simulink model "F16A_Physical"  (R2026a)
settings: Solver=VariableStepAuto
settings Model: DataDictionary=F16A_Physical.sldd  Creator=sdarshan  LastModifiedBy=sdarshan

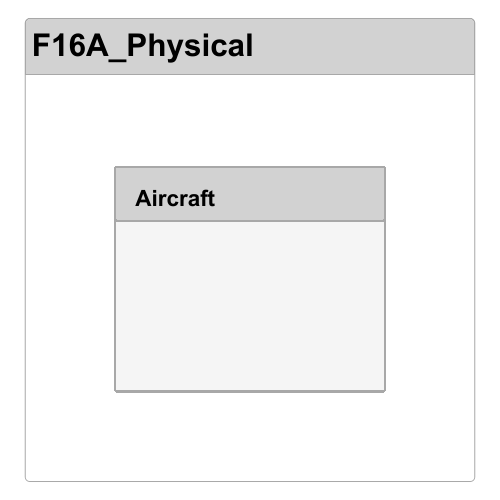
[thumbnail: Simulink's stored preview of the top-level diagram]
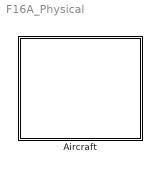
== system F16A_Physical ==
  Aircraft : Subsystem
      settings: PortSchema="{\"entries\":[{\"content\":{\"headerSize\":26,\"margin\":15,\"minimumSpacing\":25,\"sides\":[{\"content\":{},\"type\":\"ConnectorPlacement.EquallySpacedRectSide\",\"uuid\":\"d3b47e96-cd34-4867-b19b-ea6f12f6c501\"},{\"content\":{\"side\":\"RIGHT\"},\"type\":\"ConnectorPlacement.EquallySpacedRectSide\",\"uuid\":\"f31899f4-6bb1-4e7f-8ccb-f635929855f7\"},{\"content\":{\"side\":\"TOP\"},\"type\":\"ConnectorPlacement.EquallySpacedRectSide\",\"uuid\":\"ed462e8c-3ef6-416d-9984-fe5157ecba6e\"}]},\"type\":\"ConnectorPlacement.EquallySpacedConnector\",\"uuid\":\"a2af02c0-f4ca-4ebf-bacd-a22322d9a8f7\"}],\"packageUris\":[\"http://schema.mathworks.com/mf0/Connector/R2020b\"],\"version\":\"1.0\"}"

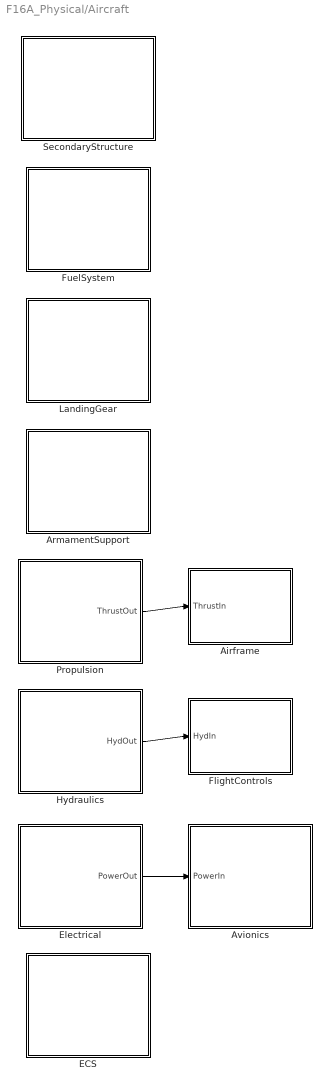
== system F16A_Physical/Aircraft ==
  Airframe : Subsystem  Variant=on  VariantControlMode=label  LabelModeActiveChoice=BlendedCrankedDelta
      settings: PortSchema="{\"entries\":[{\"content\":{\"headerSize\":38,\"margin\":15,\"minimumSpacing\":25,\"sides\":[{\"content\":{\"connectorIds\":[\"In1\"]},\"type\":\"ConnectorPlacement.EquallySpacedRectSide\",\"uuid\":\"40d085b4-dd18-4f67-ae88-aae7a5f696f7\"},{\"content\":{\"side\":\"RIGHT\"},\"type\":\"ConnectorPlacement.EquallySpacedRectSide\",\"uuid\":\"76a332b8-14bd-4810-ada5-8ab9c92fb4f5\"},{\"content\":{\"side\":\"TOP\"},\"type\":\"ConnectorPlacement.EquallySpacedRectSide\",\"uuid\":\"bda9a994-942d-4bdd-88a0-27c205fdec70\"}]},\"type\":\"ConnectorPlacement.EquallySpacedConnector\",\"uuid\":\"d2fd6e79-2d14-4962-a171-8f8cd008b298\"}],\"packageUris\":[\"http://schema.mathworks.com/mf0/Connector/R2020b\"],\"version\":\"1.0\"}"
  ArmamentSupport : Subsystem
      settings: PortSchema="{\"entries\":[{\"content\":{\"headerSize\":26,\"margin\":15,\"minimumSpacing\":25,\"sides\":[{\"content\":{},\"type\":\"ConnectorPlacement.EquallySpacedRectSide\",\"uuid\":\"d3b47e96-cd34-4867-b19b-ea6f12f6c501\"},{\"content\":{\"side\":\"RIGHT\"},\"type\":\"ConnectorPlacement.EquallySpacedRectSide\",\"uuid\":\"f31899f4-6bb1-4e7f-8ccb-f635929855f7\"},{\"content\":{\"side\":\"TOP\"},\"type\":\"ConnectorPlacement.EquallySpacedRectSide\",\"uuid\":\"ed462e8c-3ef6-416d-9984-fe5157ecba6e\"}]},\"type\":\"ConnectorPlacement.EquallySpacedConnector\",\"uuid\":\"a2af02c0-f4ca-4ebf-bacd-a22322d9a8f7\"}],\"packageUris\":[\"http://schema.mathworks.com/mf0/Connector/R2020b\"],\"version\":\"1.0\"}"
  Avionics : Subsystem
      settings: PortSchema="{\"entries\":[{\"content\":{\"headerSize\":26,\"margin\":15,\"minimumSpacing\":25,\"sides\":[{\"content\":{\"connectorIds\":[\"In1\"]},\"type\":\"ConnectorPlacement.EquallySpacedRectSide\",\"uuid\":\"d3b47e96-cd34-4867-b19b-ea6f12f6c501\"},{\"content\":{\"side\":\"RIGHT\"},\"type\":\"ConnectorPlacement.EquallySpacedRectSide\",\"uuid\":\"f31899f4-6bb1-4e7f-8ccb-f635929855f7\"},{\"content\":{\"side\":\"TOP\"},\"type\":\"ConnectorPlacement.EquallySpacedRectSide\",\"uuid\":\"ed462e8c-3ef6-416d-9984-fe5157ecba6e\"}]},\"type\":\"ConnectorPlacement.EquallySpacedConnector\",\"uuid\":\"a2af02c0-f4ca-4ebf-bacd-a22322d9a8f7\"}],\"packageUris\":[\"http://schema.mathworks.com/mf0/Connector/R2020b\"],\"version\":\"1.0\"}"
  ECS : Subsystem
      settings: PortSchema="{\"entries\":[{\"content\":{\"headerSize\":26,\"margin\":15,\"minimumSpacing\":25,\"sides\":[{\"content\":{},\"type\":\"ConnectorPlacement.EquallySpacedRectSide\",\"uuid\":\"d3b47e96-cd34-4867-b19b-ea6f12f6c501\"},{\"content\":{\"side\":\"RIGHT\"},\"type\":\"ConnectorPlacement.EquallySpacedRectSide\",\"uuid\":\"f31899f4-6bb1-4e7f-8ccb-f635929855f7\"},{\"content\":{\"side\":\"TOP\"},\"type\":\"ConnectorPlacement.EquallySpacedRectSide\",\"uuid\":\"ed462e8c-3ef6-416d-9984-fe5157ecba6e\"}]},\"type\":\"ConnectorPlacement.EquallySpacedConnector\",\"uuid\":\"a2af02c0-f4ca-4ebf-bacd-a22322d9a8f7\"}],\"packageUris\":[\"http://schema.mathworks.com/mf0/Connector/R2020b\"],\"version\":\"1.0\"}"
  Electrical : Subsystem
      settings: PortSchema="{\"entries\":[{\"content\":{\"headerSize\":26,\"margin\":15,\"minimumSpacing\":25,\"sides\":[{\"content\":{},\"type\":\"ConnectorPlacement.EquallySpacedRectSide\",\"uuid\":\"d3b47e96-cd34-4867-b19b-ea6f12f6c501\"},{\"content\":{\"connectorIds\":[\"Out1\"],\"side\":\"RIGHT\"},\"type\":\"ConnectorPlacement.EquallySpacedRectSide\",\"uuid\":\"f31899f4-6bb1-4e7f-8ccb-f635929855f7\"},{\"content\":{\"side\":\"TOP\"},\"type\":\"ConnectorPlacement.EquallySpacedRectSide\",\"uuid\":\"ed462e8c-3ef6-416d-9984-fe5157ecba6e\"}]},\"type\":\"ConnectorPlacement.EquallySpacedConnector\",\"uuid\":\"a2af02c0-f4ca-4ebf-bacd-a22322d9a8f7\"}],\"packageUris\":[\"http://schema.mathworks.com/mf0/Connector/R2020b\"],\"version\":\"1.0\"}"
  FlightControls : Subsystem  Variant=on  VariantControlMode=label  LabelModeActiveChoice=FlyByWire
      settings: PortSchema="{\"entries\":[{\"content\":{\"headerSize\":38,\"margin\":15,\"minimumSpacing\":25,\"sides\":[{\"content\":{\"connectorIds\":[\"In1\"]},\"type\":\"ConnectorPlacement.EquallySpacedRectSide\",\"uuid\":\"40d085b4-dd18-4f67-ae88-aae7a5f696f7\"},{\"content\":{\"side\":\"RIGHT\"},\"type\":\"ConnectorPlacement.EquallySpacedRectSide\",\"uuid\":\"76a332b8-14bd-4810-ada5-8ab9c92fb4f5\"},{\"content\":{\"side\":\"TOP\"},\"type\":\"ConnectorPlacement.EquallySpacedRectSide\",\"uuid\":\"bda9a994-942d-4bdd-88a0-27c205fdec70\"}]},\"type\":\"ConnectorPlacement.EquallySpacedConnector\",\"uuid\":\"d2fd6e79-2d14-4962-a171-8f8cd008b298\"}],\"packageUris\":[\"http://schema.mathworks.com/mf0/Connector/R2020b\"],\"version\":\"1.0\"}"
  FuelSystem : Subsystem
      settings: PortSchema="{\"entries\":[{\"content\":{\"headerSize\":26,\"margin\":15,\"minimumSpacing\":25,\"sides\":[{\"content\":{},\"type\":\"ConnectorPlacement.EquallySpacedRectSide\",\"uuid\":\"d3b47e96-cd34-4867-b19b-ea6f12f6c501\"},{\"content\":{\"side\":\"RIGHT\"},\"type\":\"ConnectorPlacement.EquallySpacedRectSide\",\"uuid\":\"f31899f4-6bb1-4e7f-8ccb-f635929855f7\"},{\"content\":{\"side\":\"TOP\"},\"type\":\"ConnectorPlacement.EquallySpacedRectSide\",\"uuid\":\"ed462e8c-3ef6-416d-9984-fe5157ecba6e\"}]},\"type\":\"ConnectorPlacement.EquallySpacedConnector\",\"uuid\":\"a2af02c0-f4ca-4ebf-bacd-a22322d9a8f7\"}],\"packageUris\":[\"http://schema.mathworks.com/mf0/Connector/R2020b\"],\"version\":\"1.0\"}"
  Hydraulics : Subsystem
      settings: PortSchema="{\"entries\":[{\"content\":{\"headerSize\":26,\"margin\":15,\"minimumSpacing\":25,\"sides\":[{\"content\":{},\"type\":\"ConnectorPlacement.EquallySpacedRectSide\",\"uuid\":\"d3b47e96-cd34-4867-b19b-ea6f12f6c501\"},{\"content\":{\"connectorIds\":[\"Out1\"],\"side\":\"RIGHT\"},\"type\":\"ConnectorPlacement.EquallySpacedRectSide\",\"uuid\":\"f31899f4-6bb1-4e7f-8ccb-f635929855f7\"},{\"content\":{\"side\":\"TOP\"},\"type\":\"ConnectorPlacement.EquallySpacedRectSide\",\"uuid\":\"ed462e8c-3ef6-416d-9984-fe5157ecba6e\"}]},\"type\":\"ConnectorPlacement.EquallySpacedConnector\",\"uuid\":\"a2af02c0-f4ca-4ebf-bacd-a22322d9a8f7\"}],\"packageUris\":[\"http://schema.mathworks.com/mf0/Connector/R2020b\"],\"version\":\"1.0\"}"
  LandingGear : Subsystem
      settings: PortSchema="{\"entries\":[{\"content\":{\"headerSize\":26,\"margin\":15,\"minimumSpacing\":25,\"sides\":[{\"content\":{},\"type\":\"ConnectorPlacement.EquallySpacedRectSide\",\"uuid\":\"d3b47e96-cd34-4867-b19b-ea6f12f6c501\"},{\"content\":{\"side\":\"RIGHT\"},\"type\":\"ConnectorPlacement.EquallySpacedRectSide\",\"uuid\":\"f31899f4-6bb1-4e7f-8ccb-f635929855f7\"},{\"content\":{\"side\":\"TOP\"},\"type\":\"ConnectorPlacement.EquallySpacedRectSide\",\"uuid\":\"ed462e8c-3ef6-416d-9984-fe5157ecba6e\"}]},\"type\":\"ConnectorPlacement.EquallySpacedConnector\",\"uuid\":\"a2af02c0-f4ca-4ebf-bacd-a22322d9a8f7\"}],\"packageUris\":[\"http://schema.mathworks.com/mf0/Connector/R2020b\"],\"version\":\"1.0\"}"
  Propulsion : Subsystem
      settings: PortSchema="{\"entries\":[{\"content\":{\"headerSize\":26,\"margin\":15,\"minimumSpacing\":25,\"sides\":[{\"content\":{},\"type\":\"ConnectorPlacement.EquallySpacedRectSide\",\"uuid\":\"d3b47e96-cd34-4867-b19b-ea6f12f6c501\"},{\"content\":{\"connectorIds\":[\"Out1\"],\"side\":\"RIGHT\"},\"type\":\"ConnectorPlacement.EquallySpacedRectSide\",\"uuid\":\"f31899f4-6bb1-4e7f-8ccb-f635929855f7\"},{\"content\":{\"side\":\"TOP\"},\"type\":\"ConnectorPlacement.EquallySpacedRectSide\",\"uuid\":\"ed462e8c-3ef6-416d-9984-fe5157ecba6e\"}]},\"type\":\"ConnectorPlacement.EquallySpacedConnector\",\"uuid\":\"a2af02c0-f4ca-4ebf-bacd-a22322d9a8f7\"}],\"packageUris\":[\"http://schema.mathworks.com/mf0/Connector/R2020b\"],\"version\":\"1.0\"}"
  SecondaryStructure : Subsystem
      settings: PortSchema="{\"entries\":[{\"content\":{\"headerSize\":26,\"margin\":15,\"minimumSpacing\":25,\"sides\":[{\"content\":{},\"type\":\"ConnectorPlacement.EquallySpacedRectSide\",\"uuid\":\"d3b47e96-cd34-4867-b19b-ea6f12f6c501\"},{\"content\":{\"side\":\"RIGHT\"},\"type\":\"ConnectorPlacement.EquallySpacedRectSide\",\"uuid\":\"f31899f4-6bb1-4e7f-8ccb-f635929855f7\"},{\"content\":{\"side\":\"TOP\"},\"type\":\"ConnectorPlacement.EquallySpacedRectSide\",\"uuid\":\"ed462e8c-3ef6-416d-9984-fe5157ecba6e\"}]},\"type\":\"ConnectorPlacement.EquallySpacedConnector\",\"uuid\":\"a2af02c0-f4ca-4ebf-bacd-a22322d9a8f7\"}],\"packageUris\":[\"http://schema.mathworks.com/mf0/Connector/R2020b\"],\"version\":\"1.0\"}"
  wires:
  Electrical/1(PowerOut) -> Avionics/1(PowerIn)
  Hydraulics/1(HydOut) -> FlightControls/1(HydIn)
  Propulsion/1(ThrustOut) -> Airframe/1(ThrustIn)

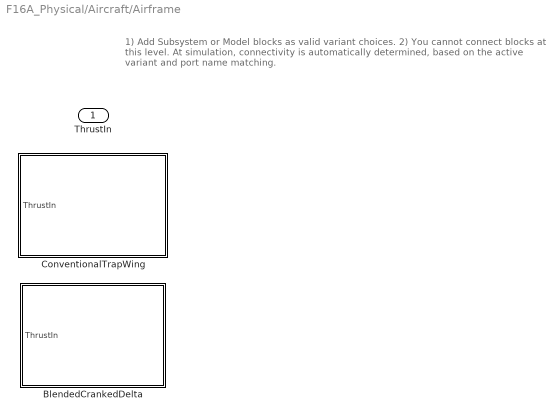
== system F16A_Physical/Aircraft/Airframe ==
  note: 1) Add Subsystem or Model blocks as valid variant choices.
      | 2) You cannot connect blocks at this level. At simulation, connectivity is automatically
      | determined, based on the active variant and port name matching.
  ThrustIn : Inport
  BlendedCrankedDelta : Subsystem  VariantControl=BlendedCrankedDelta
      settings: PortSchema="{\"entries\":[{\"content\":{\"headerSize\":26,\"margin\":15,\"minimumSpacing\":25,\"sides\":[{\"content\":{\"connectorIds\":[\"In1\"]},\"type\":\"ConnectorPlacement.EquallySpacedRectSide\",\"uuid\":\"d3b47e96-cd34-4867-b19b-ea6f12f6c501\"},{\"content\":{\"side\":\"RIGHT\"},\"type\":\"ConnectorPlacement.EquallySpacedRectSide\",\"uuid\":\"f31899f4-6bb1-4e7f-8ccb-f635929855f7\"},{\"content\":{\"side\":\"TOP\"},\"type\":\"ConnectorPlacement.EquallySpacedRectSide\",\"uuid\":\"ed462e8c-3ef6-416d-9984-fe5157ecba6e\"}]},\"type\":\"ConnectorPlacement.EquallySpacedConnector\",\"uuid\":\"a2af02c0-f4ca-4ebf-bacd-a22322d9a8f7\"}],\"packageUris\":[\"http://schema.mathworks.com/mf0/Connector/R2020b\"],\"version\":\"1.0\"}"
  ConventionalTrapWing : Subsystem  VariantControl=ConventionalTrapWing
      settings: PortSchema="{\"entries\":[{\"content\":{\"headerSize\":26,\"margin\":15,\"minimumSpacing\":25,\"sides\":[{\"content\":{\"connectorIds\":[\"In1\"]},\"type\":\"ConnectorPlacement.EquallySpacedRectSide\",\"uuid\":\"d3b47e96-cd34-4867-b19b-ea6f12f6c501\"},{\"content\":{\"side\":\"RIGHT\"},\"type\":\"ConnectorPlacement.EquallySpacedRectSide\",\"uuid\":\"f31899f4-6bb1-4e7f-8ccb-f635929855f7\"},{\"content\":{\"side\":\"TOP\"},\"type\":\"ConnectorPlacement.EquallySpacedRectSide\",\"uuid\":\"ed462e8c-3ef6-416d-9984-fe5157ecba6e\"}]},\"type\":\"ConnectorPlacement.EquallySpacedConnector\",\"uuid\":\"a2af02c0-f4ca-4ebf-bacd-a22322d9a8f7\"}],\"packageUris\":[\"http://schema.mathworks.com/mf0/Connector/R2020b\"],\"version\":\"1.0\"}"

== system F16A_Physical/Aircraft/ArmamentSupport ==

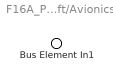
== system F16A_Physical/Aircraft/Avionics ==
  Bus Element In1 : Inport  PortName=PowerIn

== system F16A_Physical/Aircraft/ECS ==

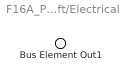
== system F16A_Physical/Aircraft/Electrical ==
  Bus Element Out1 : Outport  PortName=PowerOut

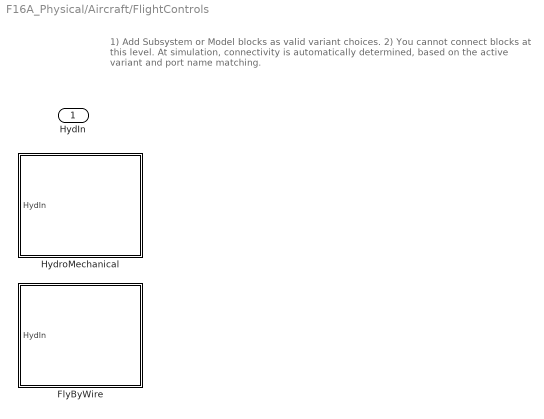
== system F16A_Physical/Aircraft/FlightControls ==
  note: 1) Add Subsystem or Model blocks as valid variant choices.
      | 2) You cannot connect blocks at this level. At simulation, connectivity is automatically
      | determined, based on the active variant and port name matching.
  HydIn : Inport
  FlyByWire : Subsystem  VariantControl=FlyByWire
      settings: PortSchema="{\"entries\":[{\"content\":{\"headerSize\":26,\"margin\":15,\"minimumSpacing\":25,\"sides\":[{\"content\":{\"connectorIds\":[\"In1\"]},\"type\":\"ConnectorPlacement.EquallySpacedRectSide\",\"uuid\":\"d3b47e96-cd34-4867-b19b-ea6f12f6c501\"},{\"content\":{\"side\":\"RIGHT\"},\"type\":\"ConnectorPlacement.EquallySpacedRectSide\",\"uuid\":\"f31899f4-6bb1-4e7f-8ccb-f635929855f7\"},{\"content\":{\"side\":\"TOP\"},\"type\":\"ConnectorPlacement.EquallySpacedRectSide\",\"uuid\":\"ed462e8c-3ef6-416d-9984-fe5157ecba6e\"}]},\"type\":\"ConnectorPlacement.EquallySpacedConnector\",\"uuid\":\"a2af02c0-f4ca-4ebf-bacd-a22322d9a8f7\"}],\"packageUris\":[\"http://schema.mathworks.com/mf0/Connector/R2020b\"],\"version\":\"1.0\"}"
  HydroMechanical : Subsystem  VariantControl=HydroMechanical
      settings: PortSchema="{\"entries\":[{\"content\":{\"headerSize\":26,\"margin\":15,\"minimumSpacing\":25,\"sides\":[{\"content\":{\"connectorIds\":[\"In1\"]},\"type\":\"ConnectorPlacement.EquallySpacedRectSide\",\"uuid\":\"d3b47e96-cd34-4867-b19b-ea6f12f6c501\"},{\"content\":{\"side\":\"RIGHT\"},\"type\":\"ConnectorPlacement.EquallySpacedRectSide\",\"uuid\":\"f31899f4-6bb1-4e7f-8ccb-f635929855f7\"},{\"content\":{\"side\":\"TOP\"},\"type\":\"ConnectorPlacement.EquallySpacedRectSide\",\"uuid\":\"ed462e8c-3ef6-416d-9984-fe5157ecba6e\"}]},\"type\":\"ConnectorPlacement.EquallySpacedConnector\",\"uuid\":\"a2af02c0-f4ca-4ebf-bacd-a22322d9a8f7\"}],\"packageUris\":[\"http://schema.mathworks.com/mf0/Connector/R2020b\"],\"version\":\"1.0\"}"

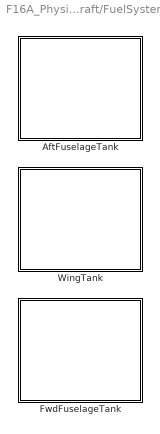
== system F16A_Physical/Aircraft/FuelSystem ==
  AftFuselageTank : Subsystem
      settings: PortSchema="{\"entries\":[{\"content\":{\"headerSize\":26,\"margin\":15,\"minimumSpacing\":25,\"sides\":[{\"content\":{},\"type\":\"ConnectorPlacement.EquallySpacedRectSide\",\"uuid\":\"d3b47e96-cd34-4867-b19b-ea6f12f6c501\"},{\"content\":{\"side\":\"RIGHT\"},\"type\":\"ConnectorPlacement.EquallySpacedRectSide\",\"uuid\":\"f31899f4-6bb1-4e7f-8ccb-f635929855f7\"},{\"content\":{\"side\":\"TOP\"},\"type\":\"ConnectorPlacement.EquallySpacedRectSide\",\"uuid\":\"ed462e8c-3ef6-416d-9984-fe5157ecba6e\"}]},\"type\":\"ConnectorPlacement.EquallySpacedConnector\",\"uuid\":\"a2af02c0-f4ca-4ebf-bacd-a22322d9a8f7\"}],\"packageUris\":[\"http://schema.mathworks.com/mf0/Connector/R2020b\"],\"version\":\"1.0\"}"
  FwdFuselageTank : Subsystem
      settings: PortSchema="{\"entries\":[{\"content\":{\"headerSize\":26,\"margin\":15,\"minimumSpacing\":25,\"sides\":[{\"content\":{},\"type\":\"ConnectorPlacement.EquallySpacedRectSide\",\"uuid\":\"d3b47e96-cd34-4867-b19b-ea6f12f6c501\"},{\"content\":{\"side\":\"RIGHT\"},\"type\":\"ConnectorPlacement.EquallySpacedRectSide\",\"uuid\":\"f31899f4-6bb1-4e7f-8ccb-f635929855f7\"},{\"content\":{\"side\":\"TOP\"},\"type\":\"ConnectorPlacement.EquallySpacedRectSide\",\"uuid\":\"ed462e8c-3ef6-416d-9984-fe5157ecba6e\"}]},\"type\":\"ConnectorPlacement.EquallySpacedConnector\",\"uuid\":\"a2af02c0-f4ca-4ebf-bacd-a22322d9a8f7\"}],\"packageUris\":[\"http://schema.mathworks.com/mf0/Connector/R2020b\"],\"version\":\"1.0\"}"
  WingTank : Subsystem
      settings: PortSchema="{\"entries\":[{\"content\":{\"headerSize\":26,\"margin\":15,\"minimumSpacing\":25,\"sides\":[{\"content\":{},\"type\":\"ConnectorPlacement.EquallySpacedRectSide\",\"uuid\":\"d3b47e96-cd34-4867-b19b-ea6f12f6c501\"},{\"content\":{\"side\":\"RIGHT\"},\"type\":\"ConnectorPlacement.EquallySpacedRectSide\",\"uuid\":\"f31899f4-6bb1-4e7f-8ccb-f635929855f7\"},{\"content\":{\"side\":\"TOP\"},\"type\":\"ConnectorPlacement.EquallySpacedRectSide\",\"uuid\":\"ed462e8c-3ef6-416d-9984-fe5157ecba6e\"}]},\"type\":\"ConnectorPlacement.EquallySpacedConnector\",\"uuid\":\"a2af02c0-f4ca-4ebf-bacd-a22322d9a8f7\"}],\"packageUris\":[\"http://schema.mathworks.com/mf0/Connector/R2020b\"],\"version\":\"1.0\"}"

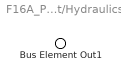
== system F16A_Physical/Aircraft/Hydraulics ==
  Bus Element Out1 : Outport  PortName=HydOut

== system F16A_Physical/Aircraft/LandingGear ==

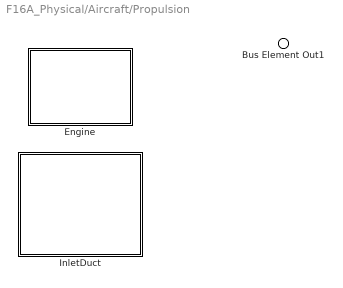
== system F16A_Physical/Aircraft/Propulsion ==
  Engine : Subsystem  Variant=on  VariantControlMode=label  LabelModeActiveChoice=F100_PW_200
      settings: PortSchema="{\"entries\":[{\"content\":{\"headerSize\":38,\"margin\":15,\"minimumSpacing\":25,\"sides\":[{\"content\":{},\"type\":\"ConnectorPlacement.EquallySpacedRectSide\",\"uuid\":\"40d085b4-dd18-4f67-ae88-aae7a5f696f7\"},{\"content\":{\"side\":\"RIGHT\"},\"type\":\"ConnectorPlacement.EquallySpacedRectSide\",\"uuid\":\"76a332b8-14bd-4810-ada5-8ab9c92fb4f5\"},{\"content\":{\"side\":\"TOP\"},\"type\":\"ConnectorPlacement.EquallySpacedRectSide\",\"uuid\":\"bda9a994-942d-4bdd-88a0-27c205fdec70\"}]},\"type\":\"ConnectorPlacement.EquallySpacedConnector\",\"uuid\":\"d2fd6e79-2d14-4962-a171-8f8cd008b298\"}],\"packageUris\":[\"http://schema.mathworks.com/mf0/Connector/R2020b\"],\"version\":\"1.0\"}"
  InletDuct : Subsystem
      settings: PortSchema="{\"entries\":[{\"content\":{\"headerSize\":26,\"margin\":15,\"minimumSpacing\":25,\"sides\":[{\"content\":{},\"type\":\"ConnectorPlacement.EquallySpacedRectSide\",\"uuid\":\"d3b47e96-cd34-4867-b19b-ea6f12f6c501\"},{\"content\":{\"side\":\"RIGHT\"},\"type\":\"ConnectorPlacement.EquallySpacedRectSide\",\"uuid\":\"f31899f4-6bb1-4e7f-8ccb-f635929855f7\"},{\"content\":{\"side\":\"TOP\"},\"type\":\"ConnectorPlacement.EquallySpacedRectSide\",\"uuid\":\"ed462e8c-3ef6-416d-9984-fe5157ecba6e\"}]},\"type\":\"ConnectorPlacement.EquallySpacedConnector\",\"uuid\":\"a2af02c0-f4ca-4ebf-bacd-a22322d9a8f7\"}],\"packageUris\":[\"http://schema.mathworks.com/mf0/Connector/R2020b\"],\"version\":\"1.0\"}"
  Bus Element Out1 : Outport  PortName=ThrustOut

== system F16A_Physical/Aircraft/SecondaryStructure ==

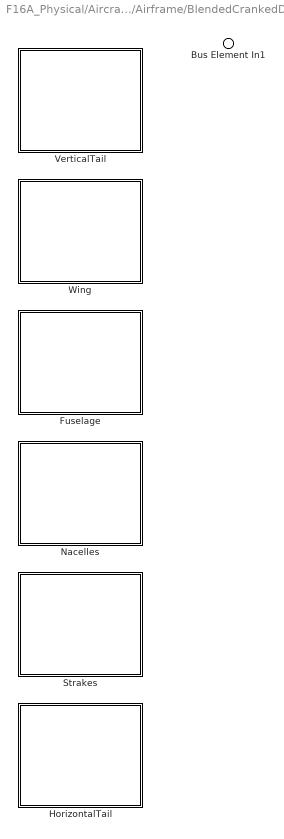
== system F16A_Physical/Aircraft/Airframe/BlendedCrankedDelta ==
  Bus Element In1 : Inport  PortName=ThrustIn
  Fuselage : Subsystem
      settings: PortSchema="{\"entries\":[{\"content\":{\"headerSize\":26,\"margin\":15,\"minimumSpacing\":25,\"sides\":[{\"content\":{},\"type\":\"ConnectorPlacement.EquallySpacedRectSide\",\"uuid\":\"d3b47e96-cd34-4867-b19b-ea6f12f6c501\"},{\"content\":{\"side\":\"RIGHT\"},\"type\":\"ConnectorPlacement.EquallySpacedRectSide\",\"uuid\":\"f31899f4-6bb1-4e7f-8ccb-f635929855f7\"},{\"content\":{\"side\":\"TOP\"},\"type\":\"ConnectorPlacement.EquallySpacedRectSide\",\"uuid\":\"ed462e8c-3ef6-416d-9984-fe5157ecba6e\"}]},\"type\":\"ConnectorPlacement.EquallySpacedConnector\",\"uuid\":\"a2af02c0-f4ca-4ebf-bacd-a22322d9a8f7\"}],\"packageUris\":[\"http://schema.mathworks.com/mf0/Connector/R2020b\"],\"version\":\"1.0\"}"
  HorizontalTail : Subsystem
      settings: PortSchema="{\"entries\":[{\"content\":{\"headerSize\":26,\"margin\":15,\"minimumSpacing\":25,\"sides\":[{\"content\":{},\"type\":\"ConnectorPlacement.EquallySpacedRectSide\",\"uuid\":\"d3b47e96-cd34-4867-b19b-ea6f12f6c501\"},{\"content\":{\"side\":\"RIGHT\"},\"type\":\"ConnectorPlacement.EquallySpacedRectSide\",\"uuid\":\"f31899f4-6bb1-4e7f-8ccb-f635929855f7\"},{\"content\":{\"side\":\"TOP\"},\"type\":\"ConnectorPlacement.EquallySpacedRectSide\",\"uuid\":\"ed462e8c-3ef6-416d-9984-fe5157ecba6e\"}]},\"type\":\"ConnectorPlacement.EquallySpacedConnector\",\"uuid\":\"a2af02c0-f4ca-4ebf-bacd-a22322d9a8f7\"}],\"packageUris\":[\"http://schema.mathworks.com/mf0/Connector/R2020b\"],\"version\":\"1.0\"}"
  Nacelles : Subsystem
      settings: PortSchema="{\"entries\":[{\"content\":{\"headerSize\":26,\"margin\":15,\"minimumSpacing\":25,\"sides\":[{\"content\":{},\"type\":\"ConnectorPlacement.EquallySpacedRectSide\",\"uuid\":\"d3b47e96-cd34-4867-b19b-ea6f12f6c501\"},{\"content\":{\"side\":\"RIGHT\"},\"type\":\"ConnectorPlacement.EquallySpacedRectSide\",\"uuid\":\"f31899f4-6bb1-4e7f-8ccb-f635929855f7\"},{\"content\":{\"side\":\"TOP\"},\"type\":\"ConnectorPlacement.EquallySpacedRectSide\",\"uuid\":\"ed462e8c-3ef6-416d-9984-fe5157ecba6e\"}]},\"type\":\"ConnectorPlacement.EquallySpacedConnector\",\"uuid\":\"a2af02c0-f4ca-4ebf-bacd-a22322d9a8f7\"}],\"packageUris\":[\"http://schema.mathworks.com/mf0/Connector/R2020b\"],\"version\":\"1.0\"}"
  Strakes : Subsystem
      settings: PortSchema="{\"entries\":[{\"content\":{\"headerSize\":26,\"margin\":15,\"minimumSpacing\":25,\"sides\":[{\"content\":{},\"type\":\"ConnectorPlacement.EquallySpacedRectSide\",\"uuid\":\"d3b47e96-cd34-4867-b19b-ea6f12f6c501\"},{\"content\":{\"side\":\"RIGHT\"},\"type\":\"ConnectorPlacement.EquallySpacedRectSide\",\"uuid\":\"f31899f4-6bb1-4e7f-8ccb-f635929855f7\"},{\"content\":{\"side\":\"TOP\"},\"type\":\"ConnectorPlacement.EquallySpacedRectSide\",\"uuid\":\"ed462e8c-3ef6-416d-9984-fe5157ecba6e\"}]},\"type\":\"ConnectorPlacement.EquallySpacedConnector\",\"uuid\":\"a2af02c0-f4ca-4ebf-bacd-a22322d9a8f7\"}],\"packageUris\":[\"http://schema.mathworks.com/mf0/Connector/R2020b\"],\"version\":\"1.0\"}"
  VerticalTail : Subsystem
      settings: PortSchema="{\"entries\":[{\"content\":{\"headerSize\":26,\"margin\":15,\"minimumSpacing\":25,\"sides\":[{\"content\":{},\"type\":\"ConnectorPlacement.EquallySpacedRectSide\",\"uuid\":\"d3b47e96-cd34-4867-b19b-ea6f12f6c501\"},{\"content\":{\"side\":\"RIGHT\"},\"type\":\"ConnectorPlacement.EquallySpacedRectSide\",\"uuid\":\"f31899f4-6bb1-4e7f-8ccb-f635929855f7\"},{\"content\":{\"side\":\"TOP\"},\"type\":\"ConnectorPlacement.EquallySpacedRectSide\",\"uuid\":\"ed462e8c-3ef6-416d-9984-fe5157ecba6e\"}]},\"type\":\"ConnectorPlacement.EquallySpacedConnector\",\"uuid\":\"a2af02c0-f4ca-4ebf-bacd-a22322d9a8f7\"}],\"packageUris\":[\"http://schema.mathworks.com/mf0/Connector/R2020b\"],\"version\":\"1.0\"}"
  Wing : Subsystem
      settings: PortSchema="{\"entries\":[{\"content\":{\"headerSize\":26,\"margin\":15,\"minimumSpacing\":25,\"sides\":[{\"content\":{},\"type\":\"ConnectorPlacement.EquallySpacedRectSide\",\"uuid\":\"d3b47e96-cd34-4867-b19b-ea6f12f6c501\"},{\"content\":{\"side\":\"RIGHT\"},\"type\":\"ConnectorPlacement.EquallySpacedRectSide\",\"uuid\":\"f31899f4-6bb1-4e7f-8ccb-f635929855f7\"},{\"content\":{\"side\":\"TOP\"},\"type\":\"ConnectorPlacement.EquallySpacedRectSide\",\"uuid\":\"ed462e8c-3ef6-416d-9984-fe5157ecba6e\"}]},\"type\":\"ConnectorPlacement.EquallySpacedConnector\",\"uuid\":\"a2af02c0-f4ca-4ebf-bacd-a22322d9a8f7\"}],\"packageUris\":[\"http://schema.mathworks.com/mf0/Connector/R2020b\"],\"version\":\"1.0\"}"

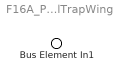
== system F16A_Physical/Aircraft/Airframe/ConventionalTrapWing ==
  Bus Element In1 : Inport  PortName=ThrustIn

== system F16A_Physical/Aircraft/FlightControls/FlyByWire ==
  Bus Element In1 : Inport  PortName=HydIn

== system F16A_Physical/Aircraft/FlightControls/HydroMechanical ==
  Bus Element In1 : Inport  PortName=HydIn

== system F16A_Physical/Aircraft/FuelSystem/AftFuselageTank ==

== system F16A_Physical/Aircraft/FuelSystem/FwdFuselageTank ==

== system F16A_Physical/Aircraft/FuelSystem/WingTank ==

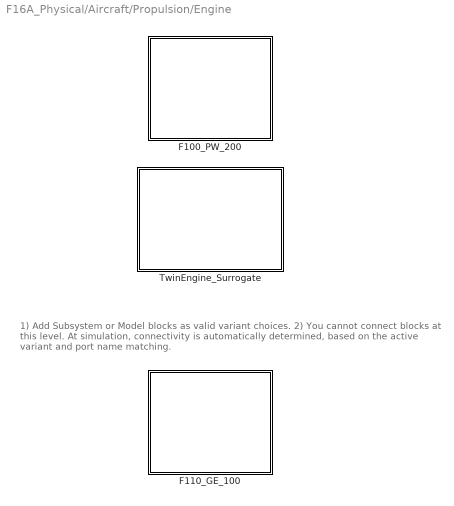
== system F16A_Physical/Aircraft/Propulsion/Engine ==
  note: 1) Add Subsystem or Model blocks as valid variant choices.
      | 2) You cannot connect blocks at this level. At simulation, connectivity is automatically
      | determined, based on the active variant and port name matching.
  F100_PW_200 : Subsystem  VariantControl=F100_PW_200
      settings: PortSchema="{\"entries\":[{\"content\":{\"headerSize\":26,\"margin\":15,\"minimumSpacing\":25,\"sides\":[{\"content\":{},\"type\":\"ConnectorPlacement.EquallySpacedRectSide\",\"uuid\":\"d3b47e96-cd34-4867-b19b-ea6f12f6c501\"},{\"content\":{\"side\":\"RIGHT\"},\"type\":\"ConnectorPlacement.EquallySpacedRectSide\",\"uuid\":\"f31899f4-6bb1-4e7f-8ccb-f635929855f7\"},{\"content\":{\"side\":\"TOP\"},\"type\":\"ConnectorPlacement.EquallySpacedRectSide\",\"uuid\":\"ed462e8c-3ef6-416d-9984-fe5157ecba6e\"}]},\"type\":\"ConnectorPlacement.EquallySpacedConnector\",\"uuid\":\"a2af02c0-f4ca-4ebf-bacd-a22322d9a8f7\"}],\"packageUris\":[\"http://schema.mathworks.com/mf0/Connector/R2020b\"],\"version\":\"1.0\"}"
  F110_GE_100 : Subsystem  VariantControl=F110_GE_100
      settings: PortSchema="{\"entries\":[{\"content\":{\"headerSize\":26,\"margin\":15,\"minimumSpacing\":25,\"sides\":[{\"content\":{},\"type\":\"ConnectorPlacement.EquallySpacedRectSide\",\"uuid\":\"d3b47e96-cd34-4867-b19b-ea6f12f6c501\"},{\"content\":{\"side\":\"RIGHT\"},\"type\":\"ConnectorPlacement.EquallySpacedRectSide\",\"uuid\":\"f31899f4-6bb1-4e7f-8ccb-f635929855f7\"},{\"content\":{\"side\":\"TOP\"},\"type\":\"ConnectorPlacement.EquallySpacedRectSide\",\"uuid\":\"ed462e8c-3ef6-416d-9984-fe5157ecba6e\"}]},\"type\":\"ConnectorPlacement.EquallySpacedConnector\",\"uuid\":\"a2af02c0-f4ca-4ebf-bacd-a22322d9a8f7\"}],\"packageUris\":[\"http://schema.mathworks.com/mf0/Connector/R2020b\"],\"version\":\"1.0\"}"
  TwinEngine_Surrogate : Subsystem  VariantControl=TwinEngine_Surrogate
      settings: PortSchema="{\"entries\":[{\"content\":{\"headerSize\":26,\"margin\":15,\"minimumSpacing\":25,\"sides\":[{\"content\":{},\"type\":\"ConnectorPlacement.EquallySpacedRectSide\",\"uuid\":\"d3b47e96-cd34-4867-b19b-ea6f12f6c501\"},{\"content\":{\"side\":\"RIGHT\"},\"type\":\"ConnectorPlacement.EquallySpacedRectSide\",\"uuid\":\"f31899f4-6bb1-4e7f-8ccb-f635929855f7\"},{\"content\":{\"side\":\"TOP\"},\"type\":\"ConnectorPlacement.EquallySpacedRectSide\",\"uuid\":\"ed462e8c-3ef6-416d-9984-fe5157ecba6e\"}]},\"type\":\"ConnectorPlacement.EquallySpacedConnector\",\"uuid\":\"a2af02c0-f4ca-4ebf-bacd-a22322d9a8f7\"}],\"packageUris\":[\"http://schema.mathworks.com/mf0/Connector/R2020b\"],\"version\":\"1.0\"}"

== system F16A_Physical/Aircraft/Propulsion/InletDuct ==

== system F16A_Physical/Aircraft/Airframe/BlendedCrankedDelta/Fuselage ==

== system F16A_Physical/Aircraft/Airframe/BlendedCrankedDelta/HorizontalTail ==

== system F16A_Physical/Aircraft/Airframe/BlendedCrankedDelta/Nacelles ==

== system F16A_Physical/Aircraft/Airframe/BlendedCrankedDelta/Strakes ==

== system F16A_Physical/Aircraft/Airframe/BlendedCrankedDelta/VerticalTail ==

== system F16A_Physical/Aircraft/Airframe/BlendedCrankedDelta/Wing ==

== system F16A_Physical/Aircraft/Propulsion/Engine/F100_PW_200 ==

== system F16A_Physical/Aircraft/Propulsion/Engine/F110_GE_100 ==

== system F16A_Physical/Aircraft/Propulsion/Engine/TwinEngine_Surrogate ==
